simulink model "PID_Controller"  (R2020b)
settings: Solver=VariableStepAuto  StartTime=0.0  StopTime=10.0  RelTol=1e-3
undefined symbols (not defined in the file or in its folder): Kd, Ki, Kp
settings Model: DataDictionary=motor_dd.sldd  Creator=Sourav Kumar  LastModifiedBy=mluser
settings DataIOCC: SaveOutput=off  SaveTime=off

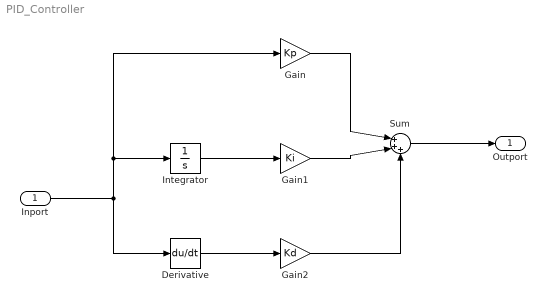
== system PID_Controller ==
  Inport : Inport  OutDataTypeStr=double  PortDimensions=1
  Derivative : Derivative
  Gain : Gain  Gain=Kp
  Gain1 : Gain  Gain=Ki
  Gain2 : Gain  Gain=Kd
  Integrator : Integrator
  Sum : Sum  Inputs=|+++
  Outport : Outport  OutDataTypeStr=double  PortDimensions=1  SampleTime=0
  wires:
  Sum/1 -> Outport/1
  Derivative/1 -> Gain2/1
  Inport/1 -> Gain/1, Integrator/1, Derivative/1
  Gain2/1 -> Sum/3
  Gain1/1 -> Sum/2
  Integrator/1 -> Gain1/1
  Gain/1 -> Sum/1
